simulink model "mdl5"  (R2014a)
settings: Solver=FixedStepDiscrete  SolverMode=SingleTasking  StartTime=TIME(1)  StopTime=TIME(end)  FixedStep=SIMSTEP  RelTol=1e-3
model workspace (MAT data in the model file):
  autoc_mdd_data01 : struct (value not decoded)
values from neighbouring files (symbols this model uses):
  map_mr4_01 = [400 500 600 700 800 900 1000 1100 1200 1300 1400 1500 ... (47 elements, 1x47)]    [scr_simdata_all.mat]
  map_mr4_02 = [0.684 0.622 0.566 0.514 0.468 0.425 0.387 0.352 0.32 0.291 0.264 0.241 ... (47 elements, 1x47)]    [scr_simdata_all.mat]
  map_mr4_03 = [10 12 14 16 18 20 22 24 26 28 30 32 ... (51 elements, 1x51)]    [scr_simdata_all.mat]
  map_mr4_04 = [0.0257 0.0124 0.00595 0.00286 0.00137 0.000662 0.000318 0.000153 7.37e-05 3.54e-05 1.7e-05 8.19e-06 ... (51 elements, 1x51)]    [scr_simdata_all.mat]
  map_mr4_05 = [10 12 14 16 18 20 22 24 26 28 30 32 ... (51 elements, 1x51)]    [scr_simdata_all.mat]
  map_mr4_06 = [0.9647 0.9835 0.9945 0.9994 0.9972 0.9871 0.97 0.9462 0.9163 0.8807 0.8403 0.796 ... (51 elements, 1x51)]    [scr_simdata_all.mat]
  map_mr4_07 = [0 1 2 3 4 5 6 7 8 9 10 11 ... (51 elements, 1x51)]    [scr_simdata_all.mat]
  map_mr4_08 = [0 0.01 0.0214 0.0335 0.0459 0.0587 0.0718 0.085 0.0985 0.112 0.126 0.14 ... (51 elements, 1x51)]    [scr_simdata_all.mat]
  Parameter114 = 126    [scr_simdata_all.mat]
  Parameter115 = 129    [scr_simdata_all.mat]
  Parameter131 = 3    [scr_simdata_all.mat]
  Parameter141 = 0    [scr_simdata_all.mat]
  Parameter143 = 1    [scr_simdata_all.mat]
  Parameter144 = 3    [scr_simdata_all.mat]
  Parameter51 = 0    [scr_simdata_all.mat]
  Parameter52 = 1    [scr_simdata_all.mat]
  Parameter53 = 2    [scr_simdata_all.mat]
  Parameter70 = 30    [scr_simdata_all.mat]
  Parameter71 = 33    [scr_simdata_all.mat]
  Parameter92 = 78    [scr_simdata_all.mat]
  Parameter93 = 81    [scr_simdata_all.mat]
  SIMSTEP = 0.0001024    [scr_simdata_all.mat]
(part 1 of 4)
Description:
  | AutoCodeGenerator:Version 1.01.A;
settings Model: autoc_cdm_savetype=ModelWorkspace  autoc_cdm_name=autoc_mdd_data01  autoc_current_model=mdl5  autoc_dsminitmode=spec  Creator=905900  LastModifiedBy=yoshi12
settings DataIOCC: SignalLoggingSaveFormat=ModelDataLogs
settings OptimizationCC: BooleanDataType=off  InlineParams=on  InlineInvariantSignals=on  ExpressionDepthLimit=2147483647  UseTempVars=on  InitFltsAndDblsToZero=on  OptimizeModelRefInitCode=on  LifeSpan=1
settings DebuggingCC: SignalInfNanChecking=warning  SaveWithParameterizedLinksMsg=none  UnderspecifiedInitializationDetection=Classic  CheckExecutionContextPreStartOutputMsg=on  CheckExecutionContextRuntimeOutputMsg=on  TimeAdjustmentMsg=warning  SolverPrmCheckMsg=none  InheritedTsInSrcMsg=none  MultiTaskDSMMsg=warning  MultiTaskCondExecSysMsg=none  TasksWithSamePriorityMsg=none  FcnCallInpInsideContextMsg=UseLocalSettings  UnconnectedInputMsg=error  UnconnectedOutputMsg=error  UnconnectedLineMsg=error  UniqueDataStoreMsg=error  BusObjectLabelMismatch=error  RootOutportRequireBusObject=error  ModelReferenceIOMsg=warning  ModelReferenceVersionMismatchMessage=warning  ModelReferenceIOMismatchMessage=warning  StateNameClashWarn=warning
settings HardwareCC: ProdIntDivRoundTo=Floor  ProdEndianess=LittleEndian  ProdHWDeviceType=Specified  TargetHWDeviceType=32-bit Generic  ProdEqTarget=off
settings ModelReferenceCC: ModelReferenceNumInstancesAllowed=Single
settings SFSimCC: SimParseCustomCode=off
settings RTWCC: SystemTargetFile=ert.tlc  GenCodeOnly=on  TemplateMakefile=ert_default_tmf  Description=Real-Time Workshop Embedded Coder (no auto configuration)  RTWVerbose=off  ProcessScript=ert_make_rtw_hook
settings CodeAppCC: ForceParamTrailComments=on  IgnoreCustomStorageClasses=off  CustomSymbolStrType=$N$R$M  InternalIdentifier=Classic
settings ERTTargetCC: TargetFcnLib=ansi_tfl_tmw.mat  ParMdlRefBuildCompliant=on  CompOptLevelCompliant=on  ConcurrentExecutionCompliant=on  ERTFirstTimeCompliant=on  ModelStepFunctionPrototypeControlCompliant=on  CPPClassGenCompliant=on  ERTCustomFileTemplate=example_file_process.tlc

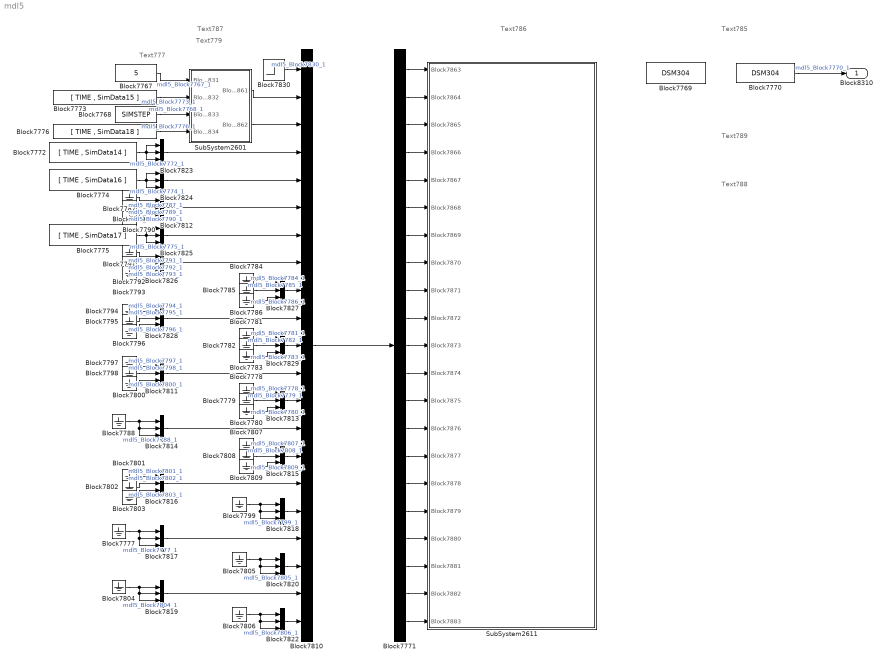
== system mdl5 ==
  note: Text789
  note: Text788
  note: Text787
  note: Text786
  note: Text785
  note: Text779
  note: Text777
  Block7767 : Constant  Value=5  OutDataTypeStr=double  SampleTime=-1
  Block7768 : Constant  Value=SIMSTEP  OutDataTypeStr=double  SampleTime=-1
  Block7769 : DataStoreMemory  DataStoreName=DSM304  InitialValue=[0 0 0]  OutDataTypeStr=double
  Block7770 : DataStoreRead  DataStoreName=DSM304
  Block7771 : Demux  Outputs=21
  Block7772 : FromWorkspace  VariableName=[ TIME , SimData14 ]  SampleTime=SIMSTEP  Interpolate=off  OutputAfterFinalValue=Holding final value
  Block7773 : FromWorkspace  VariableName=[ TIME , SimData15 ]  SampleTime=SIMSTEP  Interpolate=off  OutputAfterFinalValue=Holding final value
  Block7774 : FromWorkspace  VariableName=[ TIME , SimData16 ]  SampleTime=SIMSTEP  Interpolate=off  OutputAfterFinalValue=Holding final value
  Block7775 : FromWorkspace  VariableName=[ TIME , SimData17 ]  SampleTime=SIMSTEP  Interpolate=off  OutputAfterFinalValue=Holding final value
  Block7776 : FromWorkspace  VariableName=[ TIME , SimData18 ]  SampleTime=SIMSTEP  Interpolate=off  OutputAfterFinalValue=Holding final value
  Block{7777..7809} (33 alike) : Ground
  Block7810 : Mux  Inputs=21
  Block{7811..7820,7822..7829} (18 alike) : Mux  Inputs=3
  Block7830 : Step  Time=SIMSTEP  SampleTime=SIMSTEP
  SubSystem2601 : Subsystem
  SubSystem2611 : Subsystem
  Block8310 : Outport
  wires:
  Block7770/1 -> Block8310/1  "mdl5_Block7770_1"
  Block7810/1 -> Block7771/1
  Block7771/1 -> SubSystem2611/1(Block7863)
  Block7771/2 -> SubSystem2611/2(Block7864)
  Block7771/3 -> SubSystem2611/3(Block7865)
  Block7771/4 -> SubSystem2611/4(Block7866)
  Block7771/5 -> SubSystem2611/5(Block7867)
  Block7771/6 -> SubSystem2611/6(Block7868)
  Block7771/7 -> SubSystem2611/7(Block7869)
  Block7771/8 -> SubSystem2611/8(Block7870)
  Block7771/9 -> SubSystem2611/9(Block7871)
  Block7771/10 -> SubSystem2611/10(Block7872)
  Block7771/11 -> SubSystem2611/11(Block7873)
  Block7771/12 -> SubSystem2611/12(Block7874)
  Block7771/13 -> SubSystem2611/13(Block7875)
  Block7771/14 -> SubSystem2611/14(Block7876)
  Block7771/15 -> SubSystem2611/15(Block7877)
  Block7771/16 -> SubSystem2611/16(Block7878)
  Block7771/17 -> SubSystem2611/17(Block7879)
  Block7771/18 -> SubSystem2611/18(Block7880)
  Block7771/19 -> SubSystem2611/19(Block7881)
  Block7771/20 -> SubSystem2611/20(Block7882)
  Block7771/21 -> SubSystem2611/21(Block7883)
  Block7823/1 -> Block7810/4
  Block7772/1 -> Block7823/2, Block7823/1, Block7823/3  "mdl5_Block7772_1"
  Block7774/1 -> Block7824/3, Block7824/1, Block7824/2  "mdl5_Block7774_1"
  Block7824/1 -> Block7810/5
  Block7787/1 -> Block7812/1  "mdl5_Block7787_1"
  Block7789/1 -> Block7812/2  "mdl5_Block7789_1"
  Block7790/1 -> Block7812/3  "mdl5_Block7790_1"
  Block7812/1 -> Block7810/6
  Block7775/1 -> Block7825/3, Block7825/1, Block7825/2  "mdl5_Block7775_1"
  Block7825/1 -> Block7810/7
  Block7791/1 -> Block7826/1  "mdl5_Block7791_1"
  Block7792/1 -> Block7826/2  "mdl5_Block7792_1"
  Block7793/1 -> Block7826/3  "mdl5_Block7793_1"
  Block7826/1 -> Block7810/8
  Block7784/1 -> Block7827/1  "mdl5_Block7784_1"
  Block7785/1 -> Block7827/2  "mdl5_Block7785_1"
  Block7786/1 -> Block7827/3  "mdl5_Block7786_1"
  Block7827/1 -> Block7810/9
  Block7794/1 -> Block7828/1  "mdl5_Block7794_1"
  Block7795/1 -> Block7828/2  "mdl5_Block7795_1"
  Block7796/1 -> Block7828/3  "mdl5_Block7796_1"
  Block7828/1 -> Block7810/10
  Block7781/1 -> Block7829/1  "mdl5_Block7781_1"
  Block7782/1 -> Block7829/2  "mdl5_Block7782_1"
  Block7783/1 -> Block7829/3  "mdl5_Block7783_1"
  Block7829/1 -> Block7810/11
  Block7797/1 -> Block7811/1  "mdl5_Block7797_1"
  Block7798/1 -> Block7811/2  "mdl5_Block7798_1"
  Block7800/1 -> Block7811/3  "mdl5_Block7800_1"
  Block7811/1 -> Block7810/12
  Block7778/1 -> Block7813/1  "mdl5_Block7778_1"
  Block7779/1 -> Block7813/2  "mdl5_Block7779_1"
  Block7780/1 -> Block7813/3  "mdl5_Block7780_1"
  Block7813/1 -> Block7810/13
  Block7788/1 -> Block7814/3, Block7814/2, Block7814/1  "mdl5_Block7788_1"
  Block7814/1 -> Block7810/14
  Block7807/1 -> Block7815/1  "mdl5_Block7807_1"
  Block7808/1 -> Block7815/2  "mdl5_Block7808_1"
  Block7809/1 -> Block7815/3  "mdl5_Block7809_1"
  Block7815/1 -> Block7810/15
  Block7801/1 -> Block7816/1  "mdl5_Block7801_1"
  Block7802/1 -> Block7816/2  "mdl5_Block7802_1"
  Block7803/1 -> Block7816/3  "mdl5_Block7803_1"
  Block7816/1 -> Block7810/16
  Block7777/1 -> Block7817/3, Block7817/2, Block7817/1  "mdl5_Block7777_1"
  Block7817/1 -> Block7810/18
  Block7799/1 -> Block7818/1, Block7818/2, Block7818/3  "mdl5_Block7799_1"
  Block7818/1 -> Block7810/17
  Block7804/1 -> Block7819/3, Block7819/2, Block7819/1  "mdl5_Block7804_1"
  Block7819/1 -> Block7810/20
  Block7805/1 -> Block7820/1, Block7820/2, Block7820/3  "mdl5_Block7805_1"
  Block7820/1 -> Block7810/19
  Block7806/1 -> Block7822/3, Block7822/2, Block7822/1  "mdl5_Block7806_1"
  Block7822/1 -> Block7810/21
  Block7830/1 -> Block7810/1  "mdl5_Block7830_1"
  SubSystem2601/1(Block7861) -> Block7810/2
  SubSystem2601/2(Block7862) -> Block7810/3
  Block7767/1 -> SubSystem2601/1(Block7831)  "mdl5_Block7767_1"
  Block7773/1 -> SubSystem2601/2(Block7832)  "mdl5_Block7773_1"
  Block7768/1 -> SubSystem2601/3(Block7833)  "mdl5_Block7768_1"
  Block7776/1 -> SubSystem2601/4(Block7834)  "mdl5_Block7776_1"

== system mdl5/SubSystem2601 ==
  note: Text717
  Block7831 : Inport
  Block7832 : Inport  Port=2
  Block7833 : Inport  Port=3
  Block7834 : Inport  Port=4
  Block7835 : Constant  Value=0  OutDataTypeStr=double  SampleTime=-1
  Block7836 : Constant  OutDataTypeStr=double  SampleTime=-1
  Block7837 : Switch  Threshold=0.5  RndMeth=Zero  SaturateOnIntegerOverflow=on  InputSameDT=on
  Block7838 : UnitDelay  SampleTime=-1
  SubSystem2602 : Subsystem
  SubSystem2603 : Subsystem
  Block7861 : Outport
  Block7862 : Outport  Port=2
  wires:
  SubSystem2603/1(Block7860) -> Block7838/1, Block7862/1, SubSystem2602/2(In2)
  Block7838/1 -> SubSystem2602/1(In1)  "mdl5_SubSystem2601_Block7838_1"
  SubSystem2602/1(Out1) -> Block7837/2
  Block7836/1 -> Block7837/1  "mdl5_SubSystem2601_Block7836_1"
  Block7835/1 -> Block7837/3  "mdl5_SubSystem2601_Block7835_1"
  Block7837/1 -> Block7861/1  "mdl5_SubSystem2601_Block7837_1"
  Block7832/1 -> SubSystem2603/2(Block7840)
  Block7833/1 -> SubSystem2603/3(Block7841)
  Block7834/1 -> SubSystem2603/4(Block7842)
  Block7831/1 -> SubSystem2603/1(Block7839)

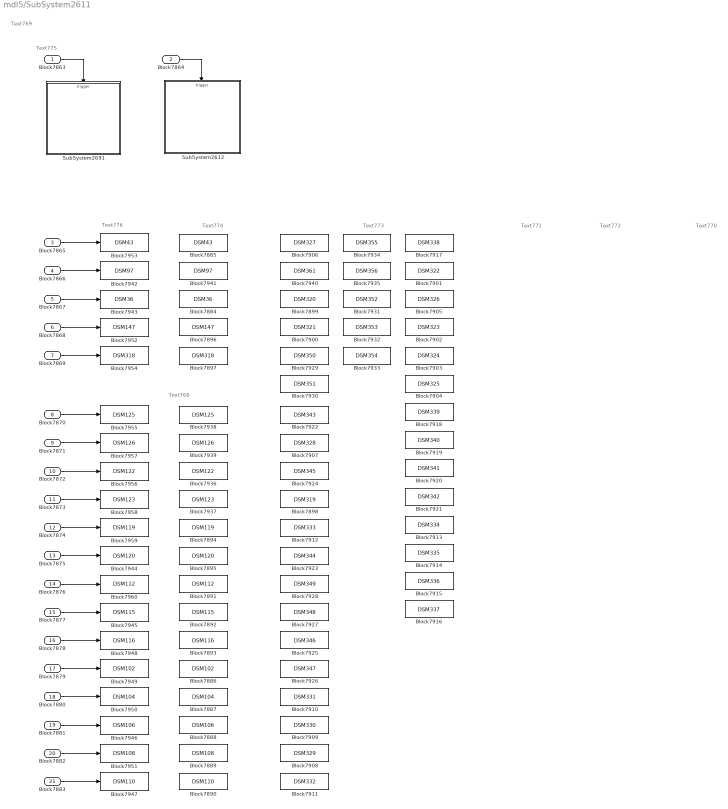
== system mdl5/SubSystem2611 ==
  note: Text776
  note: Text775
  note: Text774
  note: Text773
  note: Text772
  note: Text771
  note: Text770
  note: Text769
  note: Text768
  Block7863 : Inport
  Block7864 : Inport  Port=2
  Block7865 : Inport  Port=3
  Block7866 : Inport  Port=4
  Block7867 : Inport  Port=5
  Block7868 : Inport  Port=6
  Block7869 : Inport  Port=7
  Block7870 : Inport  Port=8
  Block7871 : Inport  Port=9
  Block7872 : Inport  Port=10
  Block7873 : Inport  Port=11
  Block7874 : Inport  Port=12
  Block7875 : Inport  Port=13
  Block7876 : Inport  Port=14
  Block7877 : Inport  Port=15
  Block7878 : Inport  Port=16
  Block7879 : Inport  Port=17
  Block7880 : Inport  Port=18
  Block7881 : Inport  Port=19
  Block7882 : Inport  Port=20
  Block7883 : Inport  Port=21
  Block7884 : DataStoreMemory  DataStoreName=DSM36  InitialValue=[0 0 0]  OutDataTypeStr=double
  Block7885 : DataStoreMemory  DataStoreName=DSM43  OutDataTypeStr=double
  Block7886 : DataStoreMemory  DataStoreName=DSM102  InitialValue=[0 0 0]  OutDataTypeStr=double
  Block7887 : DataStoreMemory  DataStoreName=DSM104  InitialValue=[0 0 0]  OutDataTypeStr=double
  Block7888 : DataStoreMemory  DataStoreName=DSM106  InitialValue=[0 0 0]  OutDataTypeStr=double
  Block7889 : DataStoreMemory  DataStoreName=DSM108  InitialValue=[0 0 0]  OutDataTypeStr=double
  Block7890 : DataStoreMemory  DataStoreName=DSM110  InitialValue=[0 0 0]  OutDataTypeStr=double
  Block7891 : DataStoreMemory  DataStoreName=DSM112  InitialValue=[0 0 0]  OutDataTypeStr=double
  Block7892 : DataStoreMemory  DataStoreName=DSM115  InitialValue=[0 0 0]  OutDataTypeStr=double
  Block7893 : DataStoreMemory  DataStoreName=DSM116  InitialValue=[0 0 0]  OutDataTypeStr=double
  Block7894 : DataStoreMemory  DataStoreName=DSM119  InitialValue=[0 0 0]  OutDataTypeStr=double
  Block7895 : DataStoreMemory  DataStoreName=DSM120  InitialValue=[0 0 0]  OutDataTypeStr=double
  Block7896 : DataStoreMemory  DataStoreName=DSM147  InitialValue=[0 0 0]  OutDataTypeStr=double
  Block7897 : DataStoreMemory  DataStoreName=DSM318  InitialValue=[0 0 0]  OutDataTypeStr=double
  Block7898 : DataStoreMemory  DataStoreName=DSM319  InitialValue=[0 0 0]  OutDataTypeStr=double
  Block7899 : DataStoreMemory  DataStoreName=DSM320  InitialValue=[0 0 0]  OutDataTypeStr=double
  Block7900 : DataStoreMemory  DataStoreName=DSM321  InitialValue=[0 0 0]  OutDataTypeStr=double
  Block7901 : DataStoreMemory  DataStoreName=DSM322  OutDataTypeStr=double
  Block7902 : DataStoreMemory  DataStoreName=DSM323  OutDataTypeStr=double
  Block7903 : DataStoreMemory  DataStoreName=DSM324  OutDataTypeStr=double
  Block7904 : DataStoreMemory  DataStoreName=DSM325  OutDataTypeStr=double
  Block7905 : DataStoreMemory  DataStoreName=DSM326  OutDataTypeStr=double
  Block7906 : DataStoreMemory  DataStoreName=DSM327  OutDataTypeStr=double
  Block7907 : DataStoreMemory  DataStoreName=DSM328  OutDataTypeStr=double
  Block7908 : DataStoreMemory  DataStoreName=DSM329  OutDataTypeStr=double
  Block7909 : DataStoreMemory  DataStoreName=DSM330  OutDataTypeStr=double
  Block7910 : DataStoreMemory  DataStoreName=DSM331  OutDataTypeStr=double
  Block7911 : DataStoreMemory  DataStoreName=DSM332  OutDataTypeStr=double
  Block7912 : DataStoreMemory  DataStoreName=DSM333  InitialValue=[0 0 0]  OutDataTypeStr=double
  Block7913 : DataStoreMemory  DataStoreName=DSM334  InitialValue=[0 0 0]  OutDataTypeStr=double
  Block7914 : DataStoreMemory  DataStoreName=DSM335  InitialValue=[0 0 0]  OutDataTypeStr=double
  Block7915 : DataStoreMemory  DataStoreName=DSM336  InitialValue=[0 0 0]  OutDataTypeStr=double
  Block7916 : DataStoreMemory  DataStoreName=DSM337  InitialValue=[0 0 0]  OutDataTypeStr=double
  Block7917 : DataStoreMemory  DataStoreName=DSM338  OutDataTypeStr=double
  Block7918 : DataStoreMemory  DataStoreName=DSM339  OutDataTypeStr=double
  Block7919 : DataStoreMemory  DataStoreName=DSM340  OutDataTypeStr=double
  Block7920 : DataStoreMemory  DataStoreName=DSM341  OutDataTypeStr=double
  Block7921 : DataStoreMemory  DataStoreName=DSM342  OutDataTypeStr=double
  Block7922 : DataStoreMemory  DataStoreName=DSM343  InitialValue=[ 0 0 0 0 0]  OutDataTypeStr=double
  Block7923 : DataStoreMemory  DataStoreName=DSM344  OutDataTypeStr=double
  Block7924 : DataStoreMemory  DataStoreName=DSM345  OutDataTypeStr=double
  Block7925 : DataStoreMemory  DataStoreName=DSM346  InitialValue=[0 0 0]  OutDataTypeStr=double
  Block7926 : DataStoreMemory  DataStoreName=DSM347  InitialValue=[0 0 0]  OutDataTypeStr=double
  Block7927 : DataStoreMemory  DataStoreName=DSM348  InitialValue=[0 0 0]  OutDataTypeStr=double
  Block7928 : DataStoreMemory  DataStoreName=DSM349  InitialValue=[0 0 0]  OutDataTypeStr=double
  Block7929 : DataStoreMemory  DataStoreName=DSM350  InitialValue=[ 0 0 0 0 0]  OutDataTypeStr=double
  Block7930 : DataStoreMemory  DataStoreName=DSM351  InitialValue=[ 0 0 0 0 0]  OutDataTypeStr=double
  Block7931 : DataStoreMemory  DataStoreName=DSM352  OutDataTypeStr=double
  Block7932 : DataStoreMemory  DataStoreName=DSM353  OutDataTypeStr=double
  Block7933 : DataStoreMemory  DataStoreName=DSM354  OutDataTypeStr=double
  Block7934 : DataStoreMemory  DataStoreName=DSM355  OutDataTypeStr=double
  Block7935 : DataStoreMemory  DataStoreName=DSM356  OutDataTypeStr=double
  Block7936 : DataStoreMemory  DataStoreName=DSM122  InitialValue=[0 0 0]  OutDataTypeStr=double
  Block7937 : DataStoreMemory  DataStoreName=DSM123  InitialValue=[0 0 0]  OutDataTypeStr=double
  Block7938 : DataStoreMemory  DataStoreName=DSM125  InitialValue=[0 0 0]  OutDataTypeStr=double
  Block7939 : DataStoreMemory  DataStoreName=DSM126  InitialValue=[0 0 0]  OutDataTypeStr=double
  Block7940 : DataStoreMemory  DataStoreName=DSM361  OutDataTypeStr=double
  Block7941 : DataStoreMemory  DataStoreName=DSM97  InitialValue=[0 0 0]  OutDataTypeStr=double
  Block7942 : DataStoreWrite  Priority=1  DataStoreName=DSM97
  Block7943 : DataStoreWrite  Priority=1  DataStoreName=DSM36
  Block7944 : DataStoreWrite  Priority=1  DataStoreName=DSM120
  Block7945 : DataStoreWrite  Priority=1  DataStoreName=DSM115
  Block7946 : DataStoreWrite  Priority=1  DataStoreName=DSM106
  Block7947 : DataStoreWrite  Priority=1  DataStoreName=DSM110
  Block7948 : DataStoreWrite  Priority=1  DataStoreName=DSM116
  Block7949 : DataStoreWrite  Priority=1  DataStoreName=DSM102
  Block7950 : DataStoreWrite  Priority=1  DataStoreName=DSM104
  Block7951 : DataStoreWrite  Priority=1  DataStoreName=DSM108
  Block7952 : DataStoreWrite  Priority=1  DataStoreName=DSM147
  Block7953 : DataStoreWrite  Priority=1  DataStoreName=DSM43
  Block7954 : DataStoreWrite  Priority=1  DataStoreName=DSM318
  Block7955 : DataStoreWrite  Priority=1  DataStoreName=DSM125
  Block7956 : DataStoreWrite  Priority=1  DataStoreName=DSM122
  Block7957 : DataStoreWrite  Priority=1  DataStoreName=DSM126
  Block7958 : DataStoreWrite  Priority=1  DataStoreName=DSM123
  Block7959 : DataStoreWrite  Priority=1  DataStoreName=DSM119
  Block7960 : DataStoreWrite  Priority=1  DataStoreName=DSM112
  SubSystem2612 : Subsystem  Priority=3  TreatAsAtomicUnit=on
      settings: AttributesFormatString=Attribute2068  RTWSystemCode=Nonreusable function  RTWFcnNameOpts=Use subsystem name
  SubSystem2691 : Subsystem  Priority=2  TreatAsAtomicUnit=on
      settings: AttributesFormatString=Attribute2129  RTWSystemCode=Nonreusable function  RTWFcnNameOpts=Use subsystem name
  wires:
  Block7864/1 -> SubSystem2612/Trigger
  Block7863/1 -> SubSystem2691/Trigger
  Block7866/1 -> Block7942/1
  Block7867/1 -> Block7943/1
  Block7865/1 -> Block7953/1
  Block7868/1 -> Block7952/1
  Block7869/1 -> Block7954/1
  Block7870/1 -> Block7955/1
  Block7871/1 -> Block7957/1
  Block7872/1 -> Block7956/1
  Block7873/1 -> Block7958/1
  Block7874/1 -> Block7959/1
  Block7875/1 -> Block7944/1
  Block7876/1 -> Block7960/1
  Block7877/1 -> Block7945/1
  Block7878/1 -> Block7948/1
  Block7879/1 -> Block7949/1
  Block7880/1 -> Block7950/1
  Block7881/1 -> Block7946/1
  Block7882/1 -> Block7951/1
  Block7883/1 -> Block7947/1

== system mdl5/SubSystem2601/SubSystem2602 ==
  note: ***編集禁止***
  In1 : Inport
  In2 : Inport  Port=2
  RO1 : RelationalOperator  Operator=~=  InputSameDT=on
  single1 : DataTypeConversion  OutDataTypeStr=single  SaturateOnIntegerOverflow=on  RndMeth=Zero
  single2 : DataTypeConversion  OutDataTypeStr=single  SaturateOnIntegerOverflow=on  RndMeth=Zero
  Out1 : Outport
  wires:
  RO1/1 -> Out1/1  "mdl5_SubSystem2601_SubSystem2602_RO1_1"
  In2/1 -> single2/1
  In1/1 -> single1/1
  single1/1 -> RO1/1  "mdl5_SubSystem2601_SubSystem2602_single1_1"
  single2/1 -> RO1/2  "mdl5_SubSystem2601_SubSystem2602_single2_1"

== system mdl5/SubSystem2601/SubSystem2603 ==
  Block7839 : Inport
  Block7840 : Inport  Port=2
  Block7841 : Inport  Port=3
  Block7842 : Inport  Port=4
  Block7843 : Constant  Value=60  OutDataTypeStr=double  SampleTime=-1
  Block7844 : Constant  Value=0  OutDataTypeStr=double  SampleTime=-1
  Block7845 : Constant  Value=360  OutDataTypeStr=double  SampleTime=-1
  Block7846 : Constant  Value=0  OutDataTypeStr=double  SampleTime=-1
  Block7847 : Constant  Value=2  OutDataTypeStr=double  SampleTime=-1
  Block7848 : Product  Inputs=**  SaturateOnIntegerOverflow=on  RndMeth=Zero  InputSameDT=on  OutDataTypeStr=Inherit: Same as first input
  Block7849 : Rounding  Operator=round
  Block7850 : Sum  Inputs=|++  OutDataTypeStr=double  RndMeth=Zero  SaturateOnIntegerOverflow=on  InputSameDT=on
  Block7851 : Switch  Threshold=0.5  RndMeth=Zero  SaturateOnIntegerOverflow=on  InputSameDT=on
  Block7852 : UnitDelay  SampleTime=-1
  Block7853 : UnitDelay  SampleTime=-1
  SubSystem2604 : Subsystem  TreatAsAtomicUnit=on  mask(***ATC.DIVISION***){bd_version=1.01.A, r0=チェック有り, r1=, r2=, r3=, r4=, r5=, r6=, r7=, r8=, r9=, c0=, c1=, c2=, c3=, c4=, c5=, c6=, c7=, c8=, c9=}
      mask prompts: bd_version "Version"
      mask help: これはAutoCからのブロックです．編集禁止．
      settings: OpenFcn=warndlg('変更禁止!');
      mask Help: web(ui_blockhelpmng(gcb));
  SubSystem2605 : Subsystem  TreatAsAtomicUnit=on  mask(***ATC.DIVISION***){bd_version=1.01.A, r0=チェック無し, r1=, r2=, r3=, r4=, r5=, r6=, r7=, r8=, r9=, c0=, c1=, c2=, c3=, c4=, c5=, c6=, c7=, c8=, c9=}
      mask prompts: bd_version "Version"
      mask help: これはAutoCからのブロックです．編集禁止．
      settings: OpenFcn=warndlg('変更禁止!');
      mask Help: web(ui_blockhelpmng(gcb));
  SubSystem2606 : Subsystem  TreatAsAtomicUnit=on  mask(***ATC.DIVISION***){bd_version=1.01.A, r0=チェック有り, r1=, r2=, r3=, r4=, r5=, r6=, r7=, r8=, r9=, c0=, c1=, c2=, c3=, c4=, c5=, c6=, c7=, c8=, c9=}
      mask prompts: bd_version "Version"
      mask help: これはAutoCからのブロックです．編集禁止．
      settings: OpenFcn=warndlg('変更禁止!');
      mask Help: web(ui_blockhelpmng(gcb));
  SubSystem2607 : Subsystem  TreatAsAtomicUnit=on  mask(***ATC.DIVISION***){bd_version=1.01.A, r0=チェック無し, r1=, r2=, r3=, r4=, r5=, r6=, r7=, r8=, r9=, c0=, c1=, c2=, c3=, c4=, c5=, c6=, c7=, c8=, c9=}
      mask prompts: bd_version "Version"
      mask help: これはAutoCからのブロックです．編集禁止．
      settings: OpenFcn=warndlg('変更禁止!');
      mask Help: web(ui_blockhelpmng(gcb));
  SubSystem2608 : Subsystem
  SubSystem2609 : Subsystem
      settings: RTWSystemCode=Inline
  Block7860 : Outport
  wires:
  Block7852/1 -> Block7850/2  "mdl5_SubSystem2601_SubSystem2603_Block7852_1"
  Block7850/1 -> Block7851/3  "mdl5_SubSystem2601_SubSystem2603_Block7850_1"
  Block7840/1 -> SubSystem2604/2(div)
  Block7844/1 -> SubSystem2604/3(init)  "mdl5_SubSystem2601_SubSystem2603_Block7844_1"
  Block7843/1 -> SubSystem2605/1(mult)  "mdl5_SubSystem2601_SubSystem2603_Block7843_1"
  SubSystem2605/1(Out) -> SubSystem2604/1(mult)
  SubSystem2606/1(Out) -> Block7850/1
  Block7841/1 -> SubSystem2606/1(mult)
  SubSystem2604/1(Out) -> SubSystem2606/2(div)
  Block7846/1 -> SubSystem2606/3(init)  "mdl5_SubSystem2601_SubSystem2603_Block7846_1"
  Block7849/1 -> Block7860/1  "mdl5_SubSystem2601_SubSystem2603_Block7849_1"
  SubSystem2608/1(Out1) -> Block7851/2
  Block7842/1 -> SubSystem2608/1(In1), Block7853/1, Block7851/1
  Block7853/1 -> SubSystem2608/2(In2)  "mdl5_SubSystem2601_SubSystem2603_Block7853_1"
  Block7851/1 -> SubSystem2609/2(Block7855)  "mdl5_SubSystem2601_SubSystem2603_Block7851_1"
  SubSystem2609/1(Block7859) -> Block7849/1, Block7852/1
  Block7845/1 -> SubSystem2607/1(mult)  "mdl5_SubSystem2601_SubSystem2603_Block7845_1"
  Block7839/1 -> SubSystem2607/2(div)
  Block7847/1 -> Block7848/2  "mdl5_SubSystem2601_SubSystem2603_Block7847_1"
  SubSystem2607/1(Out) -> SubSystem2605/2(div), Block7848/1
  Block7848/1 -> SubSystem2609/1(Block7854)  "mdl5_SubSystem2601_SubSystem2603_Block7848_1"

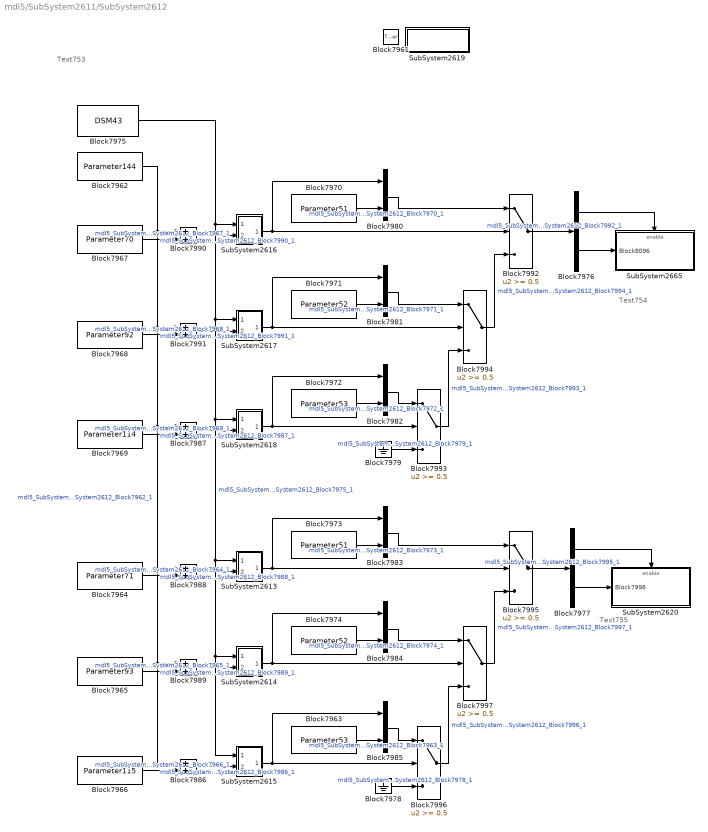
== system mdl5/SubSystem2611/SubSystem2612 ==
  note: Text755
  note: Text754
  note: Text753
  Block7961 : TriggerPort
  Block7962 : Constant  Value=Parameter144  OutDataTypeStr=double  SampleTime=-1
  Block7963 : Constant  Value=Parameter53  OutDataTypeStr=double  SampleTime=-1
  Block7964 : Constant  Value=Parameter71  OutDataTypeStr=double  SampleTime=-1
  Block7965 : Constant  Value=Parameter93  OutDataTypeStr=double  SampleTime=-1
  Block7966 : Constant  Value=Parameter115  OutDataTypeStr=double  SampleTime=-1
  Block7967 : Constant  Value=Parameter70  OutDataTypeStr=double  SampleTime=-1
  Block7968 : Constant  Value=Parameter92  OutDataTypeStr=double  SampleTime=-1
  Block7969 : Constant  Value=Parameter114  OutDataTypeStr=double  SampleTime=-1
  Block7970 : Constant  Value=Parameter51  OutDataTypeStr=double  SampleTime=-1
  Block7971 : Constant  Value=Parameter52  OutDataTypeStr=double  SampleTime=-1
  Block7972 : Constant  Value=Parameter53  OutDataTypeStr=double  SampleTime=-1
  Block7973 : Constant  Value=Parameter51  OutDataTypeStr=double  SampleTime=-1
  Block7974 : Constant  Value=Parameter52  OutDataTypeStr=double  SampleTime=-1
  Block7975 : DataStoreRead  DataStoreName=DSM43
  Block7976 : Demux  Outputs=2
  Block7977 : Demux  Outputs=2
  Block7978 : Ground
  Block7979 : Ground
  Block{7980..7985} (6 alike) : Mux  Inputs=2
  Block{7986..7991} (6 alike) : Sum  OutDataTypeStr=double  RndMeth=Zero  SaturateOnIntegerOverflow=on  InputSameDT=on
  Block{7992..7997} (6 alike) : Switch  Threshold=0.5  RndMeth=Zero  SaturateOnIntegerOverflow=on  InputSameDT=on
  SubSystem2613 : Subsystem
  SubSystem2614 : Subsystem
  SubSystem2615 : Subsystem
  SubSystem2616 : Subsystem
  SubSystem2617 : Subsystem
  SubSystem2618 : Subsystem
  SubSystem2619 : Subsystem  mask(***ATC.TriggerFunction***){}
      mask help: これはAutoCからのブロックです．編集禁止．
      settings: AttributesFormatString=Attribute2082  OpenFcn=warndlg('変更禁止!');
      mask Display: disp('ATC.Trigger Function')
  SubSystem2620 : Subsystem  TreatAsAtomicUnit=on
  SubSystem2665 : Subsystem  TreatAsAtomicUnit=on
  wires:
  Block7977/2 -> SubSystem2620/1(Block7998)
  Block7977/1 -> SubSystem2620/Enable
  Block7995/1 -> Block7977/1  "mdl5_SubSystem2611_SubSystem2612_Block7995_1"
  Block7984/1 -> Block7997/1
  Block7978/1 -> Block7996/3  "mdl5_SubSystem2611_SubSystem2612_Block7978_1"
  Block7997/1 -> Block7995/3  "mdl5_SubSystem2611_SubSystem2612_Block7997_1"
  Block7996/1 -> Block7997/3  "mdl5_SubSystem2611_SubSystem2612_Block7996_1"
  Block7963/1 -> Block7985/2  "mdl5_SubSystem2611_SubSystem2612_Block7963_1"
  Block7974/1 -> Block7984/2  "mdl5_SubSystem2611_SubSystem2612_Block7974_1"
  Block7973/1 -> Block7983/2  "mdl5_SubSystem2611_SubSystem2612_Block7973_1"
  Block7983/1 -> Block7995/1
  Block7964/1 -> Block7988/2  "mdl5_SubSystem2611_SubSystem2612_Block7964_1"
  Block7988/1 -> SubSystem2613/2(In2)  "mdl5_SubSystem2611_SubSystem2612_Block7988_1"
  Block7965/1 -> Block7989/2  "mdl5_SubSystem2611_SubSystem2612_Block7965_1"
  Block7989/1 -> SubSystem2614/2(In2)  "mdl5_SubSystem2611_SubSystem2612_Block7989_1"
  Block7966/1 -> Block7986/2  "mdl5_SubSystem2611_SubSystem2612_Block7966_1"
  Block7986/1 -> SubSystem2615/2(In2)  "mdl5_SubSystem2611_SubSystem2612_Block7986_1"
  Block7985/1 -> Block7996/1
  SubSystem2613/1(Out1) -> Block7983/1, Block7995/2
  SubSystem2614/1(Out1) -> Block7984/1, Block7997/2
  SubSystem2615/1(Out1) -> Block7985/1, Block7996/2
  Block7976/2 -> SubSystem2665/1(Block8096)
  Block7976/1 -> SubSystem2665/Enable
  Block7981/1 -> Block7994/1
  Block7979/1 -> Block7993/3  "mdl5_SubSystem2611_SubSystem2612_Block7979_1"
  Block7994/1 -> Block7992/3  "mdl5_SubSystem2611_SubSystem2612_Block7994_1"
  Block7993/1 -> Block7994/3  "mdl5_SubSystem2611_SubSystem2612_Block7993_1"
  Block7972/1 -> Block7982/2  "mdl5_SubSystem2611_SubSystem2612_Block7972_1"
  Block7971/1 -> Block7981/2  "mdl5_SubSystem2611_SubSystem2612_Block7971_1"
  Block7970/1 -> Block7980/2  "mdl5_SubSystem2611_SubSystem2612_Block7970_1"
  Block7992/1 -> Block7976/1  "mdl5_SubSystem2611_SubSystem2612_Block7992_1"
  Block7980/1 -> Block7992/1
  Block7962/1 -> Block7990/1, Block7988/1, Block7986/1, Block7989/1, Block7987/1, Block7991/1  "mdl5_SubSystem2611_SubSystem2612_Block7962_1"
  Block7967/1 -> Block7990/2  "mdl5_SubSystem2611_SubSystem2612_Block7967_1"
  Block7975/1 -> SubSystem2616/1(In1), SubSystem2613/1(In1), SubSystem2615/1(In1), SubSystem2614/1(In1), SubSystem2618/1(In1), SubSystem2617/1(In1)  "mdl5_SubSystem2611_SubSystem2612_Block7975_1"
  Block7990/1 -> SubSystem2616/2(In2)  "mdl5_SubSystem2611_SubSystem2612_Block7990_1"
  Block7968/1 -> Block7991/2  "mdl5_SubSystem2611_SubSystem2612_Block7968_1"
  Block7991/1 -> SubSystem2617/2(In2)  "mdl5_SubSystem2611_SubSystem2612_Block7991_1"
  Block7969/1 -> Block7987/2  "mdl5_SubSystem2611_SubSystem2612_Block7969_1"
  Block7987/1 -> SubSystem2618/2(In2)  "mdl5_SubSystem2611_SubSystem2612_Block7987_1"
  Block7982/1 -> Block7993/1
  SubSystem2616/1(Out1) -> Block7980/1, Block7992/2
  SubSystem2617/1(Out1) -> Block7981/1, Block7994/2
  SubSystem2618/1(Out1) -> Block7982/1, Block7993/2

== system mdl5/SubSystem2611/SubSystem2691 ==
  Block8233 : TriggerPort
  SubSystem2692 : Subsystem  mask(***ATC.TriggerFunction***){}
      mask help: これはAutoCからのブロックです．編集禁止．
      settings: AttributesFormatString=Attribute2130  OpenFcn=warndlg('変更禁止!');
      mask Display: disp('ATC.Trigger Function')
  SubSystem2693 : Subsystem  TreatAsAtomicUnit=on
      settings: AttributesFormatString=Attribute2131  RTWFcnNameOpts=Use subsystem name

== system mdl5/SubSystem2601/SubSystem2603/SubSystem2604 ==
  note: ***編集禁止***
  mult : Inport
  div : Inport  Port=2
  init : Inport  Port=3
  Product : Subsystem  TreatAsAtomicUnit=on
      settings: RTWSystemCode=Inline
  Out : Outport
  wires:
  Product/1(Out) -> Out/1
  mult/1 -> Product/1(mult)
  div/1 -> Product/2(div)
  init/1 -> Product/3(init)

== system mdl5/SubSystem2601/SubSystem2603/SubSystem2605 ==
  note: ***編集禁止***
  mult : Inport
  div : Inport  Port=2
  Product : Product  Inputs=*/  SaturateOnIntegerOverflow=on  RndMeth=Zero  InputSameDT=on  OutDataTypeStr=Inherit: Same as first input
  Out : Outport
  wires:
  Product/1 -> Out/1  "mdl5_SubSystem2601_SubSystem2603_SubSystem2605_Product_1"
  mult/1 -> Product/1
  div/1 -> Product/2

== system mdl5/SubSystem2601/SubSystem2603/SubSystem2606 ==
  note: ***編集禁止***
  mult : Inport
  div : Inport  Port=2
  init : Inport  Port=3
  Product : Subsystem  TreatAsAtomicUnit=on
      settings: RTWSystemCode=Inline
  Out : Outport
  wires:
  init/1 -> Product/3(init)
  div/1 -> Product/2(div)
  mult/1 -> Product/1(mult)
  Product/1(Out) -> Out/1

== system mdl5/SubSystem2601/SubSystem2603/SubSystem2607 ==
  note: ***編集禁止***
  mult : Inport
  div : Inport  Port=2
  Product : Product  Inputs=*/  SaturateOnIntegerOverflow=on  RndMeth=Zero  InputSameDT=on  OutDataTypeStr=Inherit: Same as first input
  Out : Outport
  wires:
  div/1 -> Product/2
  mult/1 -> Product/1
  Product/1 -> Out/1  "mdl5_SubSystem2601_SubSystem2603_SubSystem2607_Product_1"

== system mdl5/SubSystem2601/SubSystem2603/SubSystem2608 ==
  note: ***編集禁止***
  In1 : Inport
  In2 : Inport  Port=2
  RO1 : RelationalOperator  Operator=~=  InputSameDT=on
  single1 : DataTypeConversion  OutDataTypeStr=single  SaturateOnIntegerOverflow=on  RndMeth=Zero
  single2 : DataTypeConversion  OutDataTypeStr=single  SaturateOnIntegerOverflow=on  RndMeth=Zero
  Out1 : Outport
  wires:
  single2/1 -> RO1/2  "mdl5_SubSystem2601_SubSystem2603_SubSystem2608_single2_1"
  single1/1 -> RO1/1  "mdl5_SubSystem2601_SubSystem2603_SubSystem2608_single1_1"
  In1/1 -> single1/1
  In2/1 -> single2/1
  RO1/1 -> Out1/1  "mdl5_SubSystem2601_SubSystem2603_SubSystem2608_RO1_1"

== system mdl5/SubSystem2601/SubSystem2603/SubSystem2609 ==
  Block7854 : Inport
  Block7855 : Inport  Port=2
  Block7856 : Rounding  Operator=round
  Block7857 : Sum  Inputs=+-  OutDataTypeStr=double  RndMeth=Zero  SaturateOnIntegerOverflow=on  InputSameDT=on
  Block7858 : Switch  Threshold=0.5  RndMeth=Zero  SaturateOnIntegerOverflow=on  InputSameDT=on
  SubSystem2610 : Subsystem
  Block7859 : Outport
  wires:
  Block7855/1 -> Block7857/1, Block7858/3, Block7856/1
  Block7854/1 -> Block7857/2, SubSystem2610/2(In2)
  SubSystem2610/1(Out1) -> Block7858/2
  Block7858/1 -> Block7859/1  "mdl5_SubSystem2601_SubSystem2603_SubSystem2609_Block7858_1"
  Block7857/1 -> Block7858/1  "mdl5_SubSystem2601_SubSystem2603_SubSystem2609_Block7857_1"
  Block7856/1 -> SubSystem2610/1(In1)  "mdl5_SubSystem2601_SubSystem2603_SubSystem2609_Block7856_1"

== system mdl5/SubSystem2611/SubSystem2612/SubSystem2613 ==
  note: ***編集禁止***
  In1 : Inport
  In2 : Inport  Port=2
  RO1 : RelationalOperator  Operator===  InputSameDT=on
  single1 : DataTypeConversion  OutDataTypeStr=single  SaturateOnIntegerOverflow=on  RndMeth=Zero
  single2 : DataTypeConversion  OutDataTypeStr=single  SaturateOnIntegerOverflow=on  RndMeth=Zero
  Out1 : Outport
  wires:
  single2/1 -> RO1/2  "mdl5_SubSystem2611_SubSystem2612_SubSystem2613_single2_1"
  single1/1 -> RO1/1  "mdl5_SubSystem2611_SubSystem2612_SubSystem2613_single1_1"
  In1/1 -> single1/1
  In2/1 -> single2/1
  RO1/1 -> Out1/1  "mdl5_SubSystem2611_SubSystem2612_SubSystem2613_RO1_1"

== system mdl5/SubSystem2611/SubSystem2612/SubSystem2614 ==
  note: ***編集禁止***
  In1 : Inport
  In2 : Inport  Port=2
  RO1 : RelationalOperator  Operator===  InputSameDT=on
  single1 : DataTypeConversion  OutDataTypeStr=single  SaturateOnIntegerOverflow=on  RndMeth=Zero
  single2 : DataTypeConversion  OutDataTypeStr=single  SaturateOnIntegerOverflow=on  RndMeth=Zero
  Out1 : Outport
  wires:
  RO1/1 -> Out1/1  "mdl5_SubSystem2611_SubSystem2612_SubSystem2614_RO1_1"
  In2/1 -> single2/1
  In1/1 -> single1/1
  single1/1 -> RO1/1  "mdl5_SubSystem2611_SubSystem2612_SubSystem2614_single1_1"
  single2/1 -> RO1/2  "mdl5_SubSystem2611_SubSystem2612_SubSystem2614_single2_1"

== system mdl5/SubSystem2611/SubSystem2612/SubSystem2615 ==
  note: ***編集禁止***
  In1 : Inport
  In2 : Inport  Port=2
  RO1 : RelationalOperator  Operator===  InputSameDT=on
  single1 : DataTypeConversion  OutDataTypeStr=single  SaturateOnIntegerOverflow=on  RndMeth=Zero
  single2 : DataTypeConversion  OutDataTypeStr=single  SaturateOnIntegerOverflow=on  RndMeth=Zero
  Out1 : Outport
  wires:
  RO1/1 -> Out1/1  "mdl5_SubSystem2611_SubSystem2612_SubSystem2615_RO1_1"
  In2/1 -> single2/1
  In1/1 -> single1/1
  single1/1 -> RO1/1  "mdl5_SubSystem2611_SubSystem2612_SubSystem2615_single1_1"
  single2/1 -> RO1/2  "mdl5_SubSystem2611_SubSystem2612_SubSystem2615_single2_1"

== system mdl5/SubSystem2611/SubSystem2612/SubSystem2616 ==
  note: ***編集禁止***
  In1 : Inport
  In2 : Inport  Port=2
  RO1 : RelationalOperator  Operator===  InputSameDT=on
  single1 : DataTypeConversion  OutDataTypeStr=single  SaturateOnIntegerOverflow=on  RndMeth=Zero
  single2 : DataTypeConversion  OutDataTypeStr=single  SaturateOnIntegerOverflow=on  RndMeth=Zero
  Out1 : Outport
  wires:
  single2/1 -> RO1/2  "mdl5_SubSystem2611_SubSystem2612_SubSystem2616_single2_1"
  single1/1 -> RO1/1  "mdl5_SubSystem2611_SubSystem2612_SubSystem2616_single1_1"
  In1/1 -> single1/1
  In2/1 -> single2/1
  RO1/1 -> Out1/1  "mdl5_SubSystem2611_SubSystem2612_SubSystem2616_RO1_1"

== system mdl5/SubSystem2611/SubSystem2612/SubSystem2617 ==
  note: ***編集禁止***
  In1 : Inport
  In2 : Inport  Port=2
  RO1 : RelationalOperator  Operator===  InputSameDT=on
  single1 : DataTypeConversion  OutDataTypeStr=single  SaturateOnIntegerOverflow=on  RndMeth=Zero
  single2 : DataTypeConversion  OutDataTypeStr=single  SaturateOnIntegerOverflow=on  RndMeth=Zero
  Out1 : Outport
  wires:
  RO1/1 -> Out1/1  "mdl5_SubSystem2611_SubSystem2612_SubSystem2617_RO1_1"
  In2/1 -> single2/1
  In1/1 -> single1/1
  single1/1 -> RO1/1  "mdl5_SubSystem2611_SubSystem2612_SubSystem2617_single1_1"
  single2/1 -> RO1/2  "mdl5_SubSystem2611_SubSystem2612_SubSystem2617_single2_1"

== system mdl5/SubSystem2611/SubSystem2612/SubSystem2618 ==
  note: ***編集禁止***
  In1 : Inport
  In2 : Inport  Port=2
  RO1 : RelationalOperator  Operator===  InputSameDT=on
  single1 : DataTypeConversion  OutDataTypeStr=single  SaturateOnIntegerOverflow=on  RndMeth=Zero
  single2 : DataTypeConversion  OutDataTypeStr=single  SaturateOnIntegerOverflow=on  RndMeth=Zero
  Out1 : Outport
  wires:
  RO1/1 -> Out1/1  "mdl5_SubSystem2611_SubSystem2612_SubSystem2618_RO1_1"
  In2/1 -> single2/1
  In1/1 -> single1/1
  single1/1 -> RO1/1  "mdl5_SubSystem2611_SubSystem2612_SubSystem2618_single1_1"
  single2/1 -> RO1/2  "mdl5_SubSystem2611_SubSystem2612_SubSystem2618_single2_1"

== system mdl5/SubSystem2611/SubSystem2612/SubSystem2619 ==
  note: (Custom TriggerFunction)***編集禁止***<<crank144>>

== system mdl5/SubSystem2611/SubSystem2612/SubSystem2620 ==
  note: Text741
  Block7998 : Inport
  Block7999 : EnablePort
  Block8000 : Constant  OutDataTypeStr=double  SampleTime=-1
  Block8001 : Sum  OutDataTypeStr=double  RndMeth=Zero  SaturateOnIntegerOverflow=on  InputSameDT=on
  Block8002 : Sum  Inputs=++|  OutDataTypeStr=double  RndMeth=Zero  SaturateOnIntegerOverflow=on  InputSameDT=on
  SubSystem2621 : Subsystem  Priority=10  TreatAsAtomicUnit=on  mask(***ATC.DSRVEC***){bd_version=1.01.A, r0=DSM320, r1=-1, r2=, r3=, r4=, r5=, r6=, r7=, r8=, r9=, c0=, c1=, c2=, c3=, c4=, c5=, c6=, c7=, c8=, c9=}
      mask prompts: bd_version "Version"
      mask help: これはAutoCからのブロックです．編集禁止．
      settings: AttributesFormatString=Attribute2084  OpenFcn=warndlg('変更禁止!');
      mask Help: web(ui_blockhelpmng(gcb));
      mask Display: disp('ATC.DSRVEC')
  SubSystem2622 : Subsystem  Priority=10  TreatAsAtomicUnit=on  mask(***ATC.DSRVEC***){bd_version=1.01.A, r0=DSM319, r1=-1, r2=, r3=, r4=, r5=, r6=, r7=, r8=, r9=, c0=, c1=, c2=, c3=, c4=, c5=, c6=, c7=, c8=, c9=}
      mask prompts: bd_version "Version"
      mask help: これはAutoCからのブロックです．編集禁止．
      settings: AttributesFormatString=Attribute2085  OpenFcn=warndlg('変更禁止!');
      mask Help: web(ui_blockhelpmng(gcb));
      mask Display: disp('ATC.DSRVEC')
  SubSystem2623 : Subsystem  Priority=20  TreatAsAtomicUnit=on  mask(***ATC.DSWVEC***){bd_version=1.01.A, r0=DSM304, r1=-1, r2=, r3=, r4=, r5=, r6=, r7=, r8=, r9=, c0=, c1=, c2=, c3=, c4=, c5=, c6=, c7=, c8=, c9=}
      mask prompts: bd_version "Version"
      mask help: これはAutoCからのブロックです．編集禁止．
      settings: AttributesFormatString=Attribute2086  OpenFcn=warndlg('変更禁止!');
      mask Help: web(ui_blockhelpmng(gcb));
      mask Display: disp('ATC.DSRVEC')
  SubSystem2624 : Subsystem  Priority=1  TreatAsAtomicUnit=on
      settings: AttributesFormatString=Attribute2087  RTWFcnNameOpts=Use subsystem name
  wires:
  Block8002/1 -> SubSystem2622/1(element), SubSystem2621/1(element), SubSystem2623/2(element)  "mdl5_SubSystem2611_SubSystem2612_SubSystem2620_Block8002_1"
  Block8000/1 -> Block8002/2  "mdl5_SubSystem2611_SubSystem2612_SubSystem2620_Block8000_1"
  Block8001/1 -> SubSystem2623/1(input)  "mdl5_SubSystem2611_SubSystem2612_SubSystem2620_Block8001_1"
  SubSystem2622/1(Output) -> Block8001/2
  SubSystem2621/1(Output) -> Block8001/1
  Block7998/1 -> Block8002/1, SubSystem2624/1(Block8003)

== system mdl5/SubSystem2611/SubSystem2612/SubSystem2665 ==
  note: Text752
  Block8096 : Inport
  Block8097 : EnablePort
  SubSystem2666 : Subsystem  TreatAsAtomicUnit=on
      settings: AttributesFormatString=Attribute2103  RTWFcnNameOpts=Use subsystem name
  wires:
  Block8096/1 -> SubSystem2666/1(Block8098)

== system mdl5/SubSystem2611/SubSystem2691/SubSystem2692 ==
  note: (Custom TriggerFunction)***編集禁止***<<pwon>>

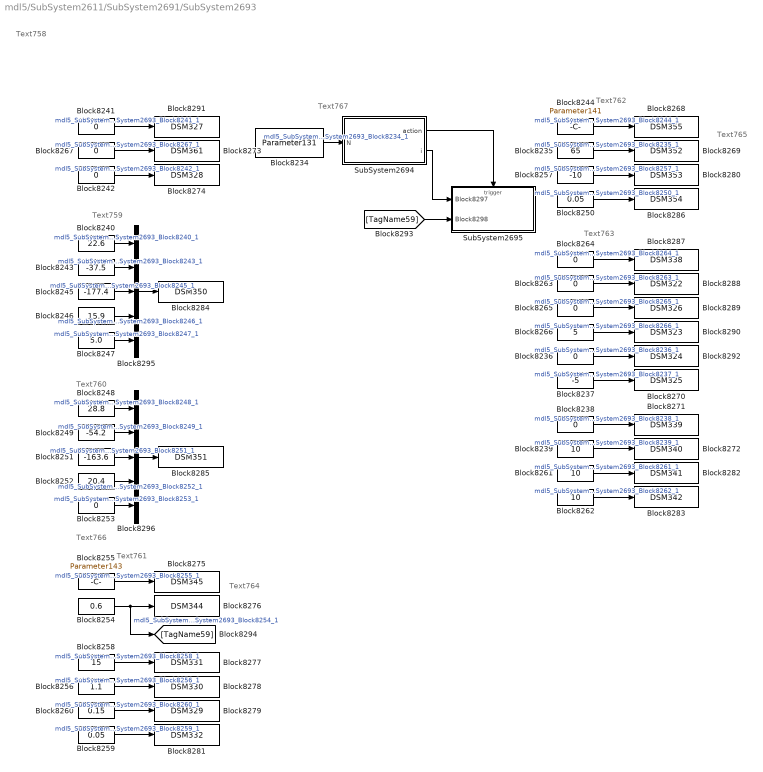
== system mdl5/SubSystem2611/SubSystem2691/SubSystem2693 ==
  note: Text767
  note: Text766
  note: Text765
  note: Text764
  note: Text763
  note: Text762
  note: Text761
  note: Text760
  note: Text759
  note: Text758
  Block8234 : Constant  Value=Parameter131  OutDataTypeStr=double  SampleTime=-1
  Block8235 : Constant  Value=65  OutDataTypeStr=double  SampleTime=-1
  Block{8236,8238,8241..8242,8253,8263..8265,8267} (9 alike) : Constant  Value=0  OutDataTypeStr=double  SampleTime=-1
  Block8237 : Constant  Value=-5  OutDataTypeStr=double  SampleTime=-1
  Block8239 : Constant  Value=10  OutDataTypeStr=double  SampleTime=-1
  Block8240 : Constant  Value=22.6  OutDataTypeStr=double  SampleTime=-1
  Block8243 : Constant  Value=-37.5  OutDataTypeStr=double  SampleTime=-1
  Block8244 : Constant  Value=Parameter141  OutDataTypeStr=double  SampleTime=-1
  Block8245 : Constant  Value=-177.4  OutDataTypeStr=double  SampleTime=-1
  Block8246 : Constant  Value=15.9  OutDataTypeStr=double  SampleTime=-1
  Block8247 : Constant  Value=5.0  OutDataTypeStr=double  SampleTime=-1
  Block8248 : Constant  Value=28.8  OutDataTypeStr=double  SampleTime=-1
  Block8249 : Constant  Value=-54.2  OutDataTypeStr=double  SampleTime=-1
  Block8250 : Constant  Value=0.05  OutDataTypeStr=double  SampleTime=-1
  Block8251 : Constant  Value=-163.6  OutDataTypeStr=double  SampleTime=-1
  Block8252 : Constant  Value=20.4  OutDataTypeStr=double  SampleTime=-1
  Block8254 : Constant  Value=0.6  OutDataTypeStr=double  SampleTime=-1
  Block8255 : Constant  Value=Parameter143  OutDataTypeStr=double  SampleTime=-1
  Block8256 : Constant  Value=1.1  OutDataTypeStr=double  SampleTime=-1
  Block8257 : Constant  Value=-10  OutDataTypeStr=double  SampleTime=-1
  Block8258 : Constant  Value=15  OutDataTypeStr=double  SampleTime=-1
  Block8259 : Constant  Value=0.05  OutDataTypeStr=double  SampleTime=-1
  Block8260 : Constant  Value=0.15  OutDataTypeStr=double  SampleTime=-1
  Block8261 : Constant  Value=10  OutDataTypeStr=double  SampleTime=-1
  Block8262 : Constant  Value=10  OutDataTypeStr=double  SampleTime=-1
  Block8266 : Constant  Value=5  OutDataTypeStr=double  SampleTime=-1
  Block8268 : DataStoreWrite  DataStoreName=DSM355
  Block8269 : DataStoreWrite  DataStoreName=DSM352
  Block8270 : DataStoreWrite  DataStoreName=DSM325
  Block8271 : DataStoreWrite  DataStoreName=DSM339
  Block8272 : DataStoreWrite  DataStoreName=DSM340
  Block8273 : DataStoreWrite  DataStoreName=DSM361
  Block8274 : DataStoreWrite  DataStoreName=DSM328
  Block8275 : DataStoreWrite  DataStoreName=DSM345
  Block8276 : DataStoreWrite  DataStoreName=DSM344
  Block8277 : DataStoreWrite  DataStoreName=DSM331
  Block8278 : DataStoreWrite  DataStoreName=DSM330
  Block8279 : DataStoreWrite  DataStoreName=DSM329
  Block8280 : DataStoreWrite  DataStoreName=DSM353
  Block8281 : DataStoreWrite  DataStoreName=DSM332
  Block8282 : DataStoreWrite  DataStoreName=DSM341
  Block8283 : DataStoreWrite  DataStoreName=DSM342
  Block8284 : DataStoreWrite  DataStoreName=DSM350
  Block8285 : DataStoreWrite  DataStoreName=DSM351
  Block8286 : DataStoreWrite  DataStoreName=DSM354
  Block8287 : DataStoreWrite  DataStoreName=DSM338
  Block8288 : DataStoreWrite  DataStoreName=DSM322
  Block8289 : DataStoreWrite  DataStoreName=DSM326
  Block8290 : DataStoreWrite  DataStoreName=DSM323
  Block8291 : DataStoreWrite  DataStoreName=DSM327
  Block8292 : DataStoreWrite  DataStoreName=DSM324
  Block8295 : Mux  Inputs=5
  Block8296 : Mux  Inputs=5
  SubSystem2694 : Subsystem  TreatAsAtomicUnit=on  mask(***ATC.ITERATOR***){}
      mask help: これはAutoCからのブロックです．編集禁止．
      settings: OpenFcn=warndlg('変更禁止!');  RTWSystemCode=Inline
  SubSystem2695 : Subsystem  TreatAsAtomicUnit=on
  wires:
  [TagName59] -> SubSystem2695/2(Block8298)
  Block8234/1 -> SubSystem2694/1(N)  "mdl5_SubSystem2611_SubSystem2691_SubSystem2693_Block8234_1"
  SubSystem2694/1(action) -> SubSystem2695/Trigger
  SubSystem2694/2(i) -> SubSystem2695/1(Block8297)
  Block8296/1 -> Block8285/1
  Block8295/1 -> Block8284/1
  Block8261/1 -> Block8282/1  "mdl5_SubSystem2611_SubSystem2691_SubSystem2693_Block8261_1"
  Block8262/1 -> Block8283/1  "mdl5_SubSystem2611_SubSystem2691_SubSystem2693_Block8262_1"
  Block8255/1 -> Block8275/1  "mdl5_SubSystem2611_SubSystem2691_SubSystem2693_Block8255_1"
  Block8254/1 -> [TagName59], Block8276/1  "mdl5_SubSystem2611_SubSystem2691_SubSystem2693_Block8254_1"
  Block8258/1 -> Block8277/1  "mdl5_SubSystem2611_SubSystem2691_SubSystem2693_Block8258_1"
  Block8256/1 -> Block8278/1  "mdl5_SubSystem2611_SubSystem2691_SubSystem2693_Block8256_1"
  Block8260/1 -> Block8279/1  "mdl5_SubSystem2611_SubSystem2691_SubSystem2693_Block8260_1"
  Block8259/1 -> Block8281/1  "mdl5_SubSystem2611_SubSystem2691_SubSystem2693_Block8259_1"
  Block8253/1 -> Block8296/5  "mdl5_SubSystem2611_SubSystem2691_SubSystem2693_Block8253_1"
  Block8252/1 -> Block8296/4  "mdl5_SubSystem2611_SubSystem2691_SubSystem2693_Block8252_1"
  Block8251/1 -> Block8296/3  "mdl5_SubSystem2611_SubSystem2691_SubSystem2693_Block8251_1"
  Block8249/1 -> Block8296/2  "mdl5_SubSystem2611_SubSystem2691_SubSystem2693_Block8249_1"
  Block8248/1 -> Block8296/1  "mdl5_SubSystem2611_SubSystem2691_SubSystem2693_Block8248_1"
  Block8247/1 -> Block8295/5  "mdl5_SubSystem2611_SubSystem2691_SubSystem2693_Block8247_1"
  Block8246/1 -> Block8295/4  "mdl5_SubSystem2611_SubSystem2691_SubSystem2693_Block8246_1"
  Block8245/1 -> Block8295/3  "mdl5_SubSystem2611_SubSystem2691_SubSystem2693_Block8245_1"
  Block8243/1 -> Block8295/2  "mdl5_SubSystem2611_SubSystem2691_SubSystem2693_Block8243_1"
  Block8241/1 -> Block8291/1  "mdl5_SubSystem2611_SubSystem2691_SubSystem2693_Block8241_1"
  Block8267/1 -> Block8273/1  "mdl5_SubSystem2611_SubSystem2691_SubSystem2693_Block8267_1"
  Block8242/1 -> Block8274/1  "mdl5_SubSystem2611_SubSystem2691_SubSystem2693_Block8242_1"
  Block8240/1 -> Block8295/1  "mdl5_SubSystem2611_SubSystem2691_SubSystem2693_Block8240_1"
  Block8244/1 -> Block8268/1  "mdl5_SubSystem2611_SubSystem2691_SubSystem2693_Block8244_1"
  Block8235/1 -> Block8269/1  "mdl5_SubSystem2611_SubSystem2691_SubSystem2693_Block8235_1"
  Block8257/1 -> Block8280/1  "mdl5_SubSystem2611_SubSystem2691_SubSystem2693_Block8257_1"
  Block8250/1 -> Block8286/1  "mdl5_SubSystem2611_SubSystem2691_SubSystem2693_Block8250_1"
  Block8264/1 -> Block8287/1  "mdl5_SubSystem2611_SubSystem2691_SubSystem2693_Block8264_1"
  Block8263/1 -> Block8288/1  "mdl5_SubSystem2611_SubSystem2691_SubSystem2693_Block8263_1"
  Block8265/1 -> Block8289/1  "mdl5_SubSystem2611_SubSystem2691_SubSystem2693_Block8265_1"
  Block8266/1 -> Block8290/1  "mdl5_SubSystem2611_SubSystem2691_SubSystem2693_Block8266_1"
  Block8236/1 -> Block8292/1  "mdl5_SubSystem2611_SubSystem2691_SubSystem2693_Block8236_1"
  Block8237/1 -> Block8270/1  "mdl5_SubSystem2611_SubSystem2691_SubSystem2693_Block8237_1"
  Block8238/1 -> Block8271/1  "mdl5_SubSystem2611_SubSystem2691_SubSystem2693_Block8238_1"
  Block8239/1 -> Block8272/1  "mdl5_SubSystem2611_SubSystem2691_SubSystem2693_Block8239_1"

== system mdl5/SubSystem2601/SubSystem2603/SubSystem2604/Product ==
  note: ***編集禁止***
  mult : Inport
  div : Inport  Port=2
  init : Inport  Port=3
  Constant1 : Constant  OutDataTypeStr=Inherit: Inherit via back propagation
  Constant2 : Constant  Value=0  OutDataTypeStr=Inherit: Inherit via back propagation
  Product : Product  Inputs=*/  SaturateOnIntegerOverflow=on  RndMeth=Zero  InputSameDT=on  OutDataTypeStr=Inherit: Same as first input
  RelationalOperator : RelationalOperator  Operator=~=  InputSameDT=on
  Switch : Switch  Threshold=0.5  SaturateOnIntegerOverflow=on  InputSameDT=on
  Switch1 : Switch  Threshold=0.5  SaturateOnIntegerOverflow=on  InputSameDT=on
  Out : Outport
  wires:
  Constant1/1 -> Switch1/3  "mdl5_SubSystem2601_SubSystem2603_SubSystem2604_Product_Constant1_1"
  Constant2/1 -> RelationalOperator/2  "mdl5_SubSystem2601_SubSystem2603_SubSystem2604_Product_Constant2_1"
  Switch1/1 -> Product/2  "mdl5_SubSystem2601_SubSystem2603_SubSystem2604_Product_Switch1_1"
  div/1 -> RelationalOperator/1, Switch1/1
  Switch/1 -> Out/1  "mdl5_SubSystem2601_SubSystem2603_SubSystem2604_Product_Switch_1"
  init/1 -> Switch/3
  RelationalOperator/1 -> Switch1/2, Switch/2  "mdl5_SubSystem2601_SubSystem2603_SubSystem2604_Product_RelationalOperator_1"
  Product/1 -> Switch/1  "mdl5_SubSystem2601_SubSystem2603_SubSystem2604_Product_Product_1"
  mult/1 -> Product/1

== system mdl5/SubSystem2601/SubSystem2603/SubSystem2606/Product ==
  note: ***編集禁止***
  mult : Inport
  div : Inport  Port=2
  init : Inport  Port=3
  Constant1 : Constant  OutDataTypeStr=Inherit: Inherit via back propagation
  Constant2 : Constant  Value=0  OutDataTypeStr=Inherit: Inherit via back propagation
  Product : Product  Inputs=*/  SaturateOnIntegerOverflow=on  RndMeth=Zero  InputSameDT=on  OutDataTypeStr=Inherit: Same as first input
  RelationalOperator : RelationalOperator  Operator=~=  InputSameDT=on
  Switch : Switch  Threshold=0.5  SaturateOnIntegerOverflow=on  InputSameDT=on
  Switch1 : Switch  Threshold=0.5  SaturateOnIntegerOverflow=on  InputSameDT=on
  Out : Outport
  wires:
  Constant1/1 -> Switch1/3  "mdl5_SubSystem2601_SubSystem2603_SubSystem2606_Product_Constant1_1"
  Constant2/1 -> RelationalOperator/2  "mdl5_SubSystem2601_SubSystem2603_SubSystem2606_Product_Constant2_1"
  Switch1/1 -> Product/2  "mdl5_SubSystem2601_SubSystem2603_SubSystem2606_Product_Switch1_1"
  div/1 -> RelationalOperator/1, Switch1/1
  Switch/1 -> Out/1  "mdl5_SubSystem2601_SubSystem2603_SubSystem2606_Product_Switch_1"
  init/1 -> Switch/3
  RelationalOperator/1 -> Switch1/2, Switch/2  "mdl5_SubSystem2601_SubSystem2603_SubSystem2606_Product_RelationalOperator_1"
  Product/1 -> Switch/1  "mdl5_SubSystem2601_SubSystem2603_SubSystem2606_Product_Product_1"
  mult/1 -> Product/1

== system mdl5/SubSystem2601/SubSystem2603/SubSystem2609/SubSystem2610 ==
  note: ***編集禁止***
  In1 : Inport
  In2 : Inport  Port=2
  LO1 : Logic  Operator=OR
  RO1 : RelationalOperator  InputSameDT=on
  RO2 : RelationalOperator  Operator===  InputSameDT=on
  single1 : DataTypeConversion  OutDataTypeStr=single  SaturateOnIntegerOverflow=on  RndMeth=Zero
  single2 : DataTypeConversion  OutDataTypeStr=single  SaturateOnIntegerOverflow=on  RndMeth=Zero
  Out1 : Outport
  wires:
  In2/1 -> single2/1
  In1/1 -> single1/1
  single1/1 -> RO1/1, RO2/1  "mdl5_SubSystem2601_SubSystem2603_SubSystem2609_SubSystem2610_single1_1"
  single2/1 -> RO1/2, RO2/2  "mdl5_SubSystem2601_SubSystem2603_SubSystem2609_SubSystem2610_single2_1"
  RO1/1 -> LO1/1  "mdl5_SubSystem2601_SubSystem2603_SubSystem2609_SubSystem2610_RO1_1"
  RO2/1 -> LO1/2  "mdl5_SubSystem2601_SubSystem2603_SubSystem2609_SubSystem2610_RO2_1"
  LO1/1 -> Out1/1  "mdl5_SubSystem2601_SubSystem2603_SubSystem2609_SubSystem2610_LO1_1"
